simulink model "Glidescope_Flare_Simulink"  (R2024b)
settings: Solver=VariableStepAuto  StartTime=0.0  StopTime=250  RelTol=1e-3
values from neighbouring files (symbols this model uses):
  A_ac_p8 = A_long_p8(1:5,1:5)    [HA_ES_MainCode.m]    (also in PitchController.mat = [0 0 0.00013165266625 3.15369085605e-06 -4.69868043887e-21 2; glidescope.mat = [0 0 0.00013165266625 3.15369085605e-06 -4.69868043887e-21 2)
  B_ac_p8 = A_long_p8(1:5,6:7)    [HA_ES_MainCode.m]    (also in PitchController.mat = [0  0; 0  0; 0.00154396044469  -0.00453382205143; -9.4930881; glidescope.mat = [0  0; 0  0; 0.00154396044469  -0.00453382205143; -9.4930881)
  C_ac_p8 = C_long_p8(1:5,1:5)    [HA_ES_MainCode.m]    (also in PitchController.mat = [1 0 0 0 0 0 57.2957795131 0 0 0 0 0 ... (25 elements, 5x5)]; glidescope.mat = [1 0 0 0 0 0 57.2957795131 0 0 0 0 0 ... (25 elements, 5x5)])
  D_ac_p8 = C_long_p8(1:5,6:7)    [HA_ES_MainCode.m]    (also in PitchController.mat = [0  0; 0  0; 0  0; 0  0; 0  0]; glidescope.mat = [0  0; 0  0; 0  0; 0  0; 0  0])
  h0 = double(sol.h0)    [HA_ES_MainCode.m]    (also in PitchController.mat = 8.35170678627; glidescope.mat = 8.35170678627)
  hf = double(sol.hf)    [HA_ES_MainCode.m]    (also in PitchController.mat = 52.4513473104; glidescope.mat = 52.4513473104)
  Kv = 100    [HA_ES_MainCode.m]    (also in PitchController.mat; glidescope.mat)
  tau = double(sol.tau)    [HA_ES_MainCode.m]    (also in PitchController.mat = 0.497; glidescope.mat = 3.34068271451)
  xu_lo = [0 0 15000 0 0.0779375118365 0 500 0.0779375118365 0 0 0 0 ... (18 elements, 18x1)]    [PitchController.mat]    (also in glidescope.mat = [0 0 5000 0 0.182405640343 0 300 0.182405640343 0 0 0 0 ... )
libraries: slpidlib x1
settings Model: Creator=henryadam  LastModifiedBy=henryadam

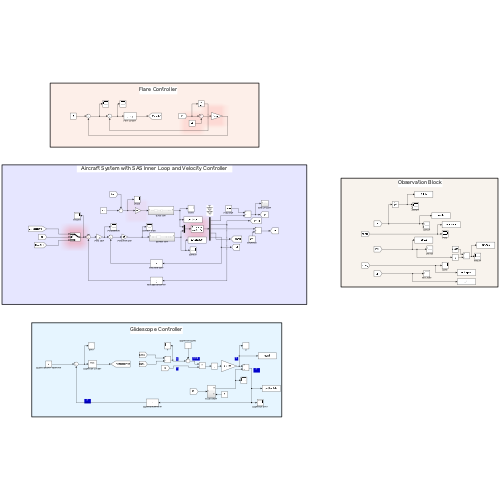
[thumbnail: Simulink's stored preview of the top-level diagram]
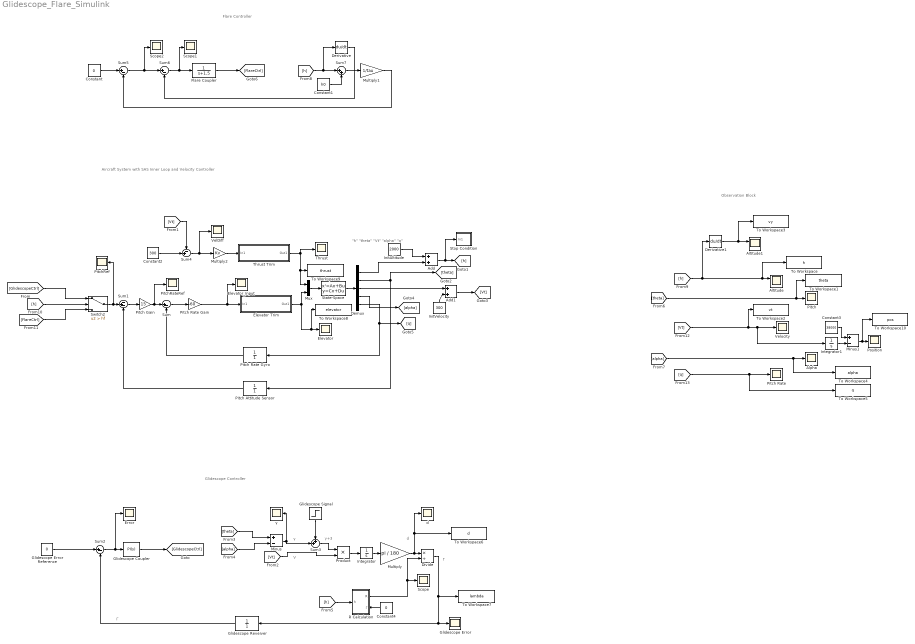
== system Glidescope_Flare_Simulink ==
  note: Aircraft System with SAS Inner Loop and Velocity Controller
  note: Glidescope Controller
  note: Flare Controller
  note: γ
  note: V
  note: Γ
  note: Γ
  note: "h"
      | "theta"
      | "Vt"
      | "alpha"
      | "q"
  note: γ+3
  note: d
  note: Observation Block
  Add : Sum
  Add1 : Sum
  Alpha : Scope
  Altitude : Scope  NumInputPorts=2
  Altitude1 : Scope  NumInputPorts=2
  Constant : Constant  Value=0
  Constant1 : Constant  Value=h0
  Constant2 : Constant  Value=300
  Constant3 : Constant  Value=38000
  Constant4 : Constant  Value=0
  Demux : Demux  Outputs=5
  Derivative : Derivative
  Derivative1 : Derivative
  Divide : Product  Inputs=*/
  Elevator : Scope
  Elevator Trim : Subsystem
  Elevator_Input : Scope
  Error : Scope
  Flare Coupler : TransferFcn  Denominator=[1 1.5]
  Glidescope Coupler : slpidlib/PID Controller  Controller=PI  Form=Parallel  TimeDomain=Continuous-time  UseExternalTs=off  SampleTime=-1  IntegratorMethod=Forward Euler  FilterMethod=Forward Euler  ControllerParametersSource=internal  P=17000  I=4000  UseKiTs=off  D=0  UseExternalDerivativeSource=off  N=100  UseFilter=on  TunerSelectOption=Transfer Function Based (PID Tuner App)  InitialConditionSource=internal  InitialConditionForIntegrator=0  InitialConditionForFilter=0  DifferentiatorICPrevScaledInput=0  ExternalReset=none  TrackingMode=off  Kt=1  LimitOutput=off  SatLimitsSource=internal  UpperSaturationLimit=inf  LowerSaturationLimit=-inf  LinearizeAsGain=on  AntiWindupMode=none  Kb=1  LimitIntegrator=off  UpperIntegratorSaturationLimit=inf  LowerIntegratorSaturationLimit=-inf  POutMin=[]  POutMax=[]  IOutMin=[]  IOutMax=[]  DOutMin=[]  DOutMax=[]  NOutMin=[]  NOutMax=[]  SumOutMin=[]  SumOutMax=[]  SaturationOutMin=[]  SaturationOutMax=[]  PParamMin=[]  PParamMax=[]  IParamMin=[]  IParamMax=[]  DParamMin=[]  DParamMax=[]  NParamMin=[]  NParamMax=[]  KbParamMin=[]  KbParamMax=[]  KtParamMin=[]  KtParamMax=[]  KbOutMin=[]  KbOutMax=[]  KtOutMin=[]  KtOutMax=[]  IntegratorOutMin=[]  IntegratorOutMax=[]  FilterOutMin=[]  FilterOutMax=[]  SumI1OutMin=[]  SumI1OutMax=[]  SumI2OutMin=[]  SumI2OutMax=[]  SumI3OutMin=[]  SumI3OutMax=[]  SumI4OutMin=[]  SumI4OutMax=[]  SumDOutMin=[]  SumDOutMax=[]  DifferentiatorOutMin=[]  DifferentiatorOutMax=[]  FilterDiffOutCoefMin=[]  FilterDiffOutCoefMax=[]  ReciprocalOutMin=[]  ReciprocalOutMax=[]  SumDenOutMin=[]  SumDenOutMax=[]  SumNumOutMin=[]  SumNumOutMax=[]  DivideOutMin=[]  DivideOutMax=[]  UdiffTsProdOutMin=[]  UdiffTsProdOutMax=[]  NTsProdOutMin=[]  NTsProdOutMax=[]  UintegralTsProdOutMin=[]  UintegralTsProdOutMax=[]  UngainTsProdOutMin=[]  UngainTsProdOutMax=[]  ClampingZeroOutDataTypeStr=Inherit: Inherit via back propagation  ClampingZeroOutMin=[]  ClampingZeroOutMax=[]  FilterDenConstantOutDataTypeStr=Inherit: Inherit via back propagation  FilterDenConstantOutMin=[]  FilterDenConstantOutMax=[]  PCopyOutDataTypeStr=Inherit: Inherit via back propagation  PCopyOutMin=[]  PCopyOutMax=[]  NCopyOutDataTypeStr=Inherit: Inherit via back propagation  NCopyOutMin=[]  NCopyOutMax=[]  IntegratorContinuousStateAttributes=''  IntegratorStateMustResolveToSignalObject=off  IntegratorRTWStateStorageClass=Auto  FilterContinuousStateAttributes=''  FilterStateMustResolveToSignalObject=off  FilterRTWStateStorageClass=Auto  ParallelPVariant=InternalParameters  IdealPVariant=Disabled  IVariant=InternalParameters  DVariant=Disabled  IntegratorVariant=Continuous  SatVariant=Disabled  AWVariant=Passthrough  PCopyVariant=Disabled  TRVariant=Disabled  FdbkBlocksVariant=Forward  IdealPFdbkVariant=Disabled  SatFdbkVariant=Disabled  DerivativeFilterVariant=Disabled  NVariant=Disabled  NCopyVariant=Disabled_SignalSpec  FilterICVariant=Disabled  IntegratorICVariant=InternalICs  ExternalResetVariant=Disabled  TRSumVariant=Passthrough  SumFdbkVariant=Disabled  SumVariant=Sum_PI  TsampFilterVariant=InternalTs  TsampNgainVariant=Passthrough  TsampIntegralVariant=Disabled_SignalSpec  ExternalSaturationOutDataTypeStr=Inherit: Same as second input  DerivativeSourceVariant=Disabled  PreIntVariant=InternalPreInt
  Glidescope Error : Scope
  Glidescope Error Reference : Constant  Value=0
  Glidescope Reveiver : TransferFcn  Denominator=[1]
  Glidescope Signal : Step  Time=10  After=3  SampleTime=0
  InitAltitude : Constant  Value=2000
  InitVelocity : Constant  Value=300
  Integrator : Integrator
  Integrator1 : Integrator
  Minus : Sum  Inputs=+-
  Minus1 : Sum  Inputs=+-
  Multiply : Gain  Gain=pi / 180
  Multiply1 : Gain  Gain=1/tau
  Multiply2 : Gain  Gain=Kv
  Mux : Mux  Inputs=2
  Pitch : Scope
  Pitch Attitude Sensor : TransferFcn  Denominator=[1]
  Pitch Gain : Gain  Gain=15
  Pitch Rate : Scope
  Pitch Rate Gain : Gain  Gain=-60
  Pitch Rate Gyro : TransferFcn  Denominator=[1]
  PitchRateRef : Scope
  PitchRef : Scope
  Position : Scope
  Product : Product
  R Calculation : Subsystem
      settings: PortSchema="{\"entries\":[{\"content\":{\"sides\":[{\"content\":{\"connectorIds\":[\"In1\"]},\"type\":\"ConnectorPlacement.EquallySpacedRectSide\",\"uuid\":\"a58ea4d3-e7df-4749-b01a-fc0a42cf2060\"},{\"content\":{\"connectorIds\":[\"Out1\",\"In2\"],\"side\":\"RIGHT\"},\"type\":\"ConnectorPlacement.EquallySpacedRectSide\",\"uuid\":\"27d5ff2b-4e59-4ac1-b665-58941cf67848\"},{\"content\":{\"side\":\"TOP\"},\"type\":\"ConnectorPlacement.EquallySpacedRectSide\",\"uuid\":\"e99417a1-aceb-4143-96dd-16120f62f201\"}]},\"type\":\"ConnectorPlacement.EquallySpacedConnector\",\"uuid\":\"f753324d-1728-43c1-b72b-a766f20cfffb\"}],\"packageUris\":[\"http://schema.mathworks.com/mf0/Connector/R2020b\"],\"version\":\"1.0\"}"
  Scope : Scope
  Scope1 : Scope
  Scope2 : Scope
  State-Space : StateSpace  A=A_ac_p8  B=B_ac_p8  C=C_ac_p8  D=D_ac_p8  InitialCondition=0
  Stop Condition : Subsystem
  Sum{,2,5..6} (4 alike) : Sum  Inputs=|+-
  Sum1 : Sum  Inputs=-+-
  Sum3 : Sum  Inputs=++|
  Sum4 : Sum  Inputs=-+|
  Sum7 : Sum  Inputs=|++
  Switch2 : Switch  Criteria=u2 > Threshold  Threshold=hf  SaturateOnIntegerOverflow=off  InputSameDT=off
  Thrust : Scope
  "Thrust Trim " : Subsystem
  To Workspace : ToWorkspace  VariableName=h  SaveFormat=Timeseries  SampleTime=-1
  To Workspace1 : ToWorkspace  VariableName=theta  SaveFormat=Timeseries  SampleTime=-1
  To Workspace10 : ToWorkspace  VariableName=pos  SaveFormat=Timeseries  SampleTime=-1
  To Workspace2 : ToWorkspace  VariableName=vt  SaveFormat=Timeseries  SampleTime=-1
  To Workspace3 : ToWorkspace  VariableName=vy  SaveFormat=Timeseries  SampleTime=-1
  To Workspace4 : ToWorkspace  VariableName=alpha  SaveFormat=Timeseries  SampleTime=-1
  To Workspace5 : ToWorkspace  VariableName=q  SaveFormat=Timeseries  SampleTime=-1
  To Workspace6 : ToWorkspace  VariableName=d  SaveFormat=Timeseries  SampleTime=-1
  To Workspace7 : ToWorkspace  VariableName=lambda  SaveFormat=Timeseries  SampleTime=-1
  To Workspace8 : ToWorkspace  VariableName=elevator  SaveFormat=Timeseries  SampleTime=-1
  To Workspace9 : ToWorkspace  VariableName=thrust  SaveFormat=Timeseries  SampleTime=-1
  VelDiff : Scope
  "Velocity " : Scope
  d : Scope
  γ : Scope
  wires:
  Sum/1 -> Pitch Rate Gain/1
  Pitch Rate Gyro/1 -> Sum/2
  Pitch Gain/1 -> PitchRateRef/1, Sum/1
  Sum1/1 -> Pitch Gain/1
  Pitch Attitude Sensor/1 -> Sum1/3
  Multiply/1 -> To Workspace6/1, d/1, Divide/1
  Divide/1 -> To Workspace7/1, Glidescope Error/1, Glidescope Reveiver/1
  Sum2/1 -> Error/1, Glidescope Coupler/1
  Pitch Rate Gain/1 -> Elevator Trim/1(In1), Elevator_Input/1
  Elevator Trim/1(Out1) -> Mux/2, To Workspace8/1, Elevator/1
  "Thrust Trim "/1(Out1) -> To Workspace9/1, Mux/1, Thrust/1
  Mux/1 -> State-Space/1
  State-Space/1 -> Demux/1
  Glidescope Error Reference/1 -> Sum2/1
  Minus/1 -> Sum3/2, γ/1
  Glidescope Signal/1 -> Sum3/1
  Sum3/1 -> Product/1
  Sum6/1 -> Scope1/1, Flare Coupler/1
  [h] -> Sum7/1, Derivative/1
  Derivative/1 -> Sum6/2
  Multiply1/1 -> Sum5/2
  Sum4/1 -> VelDiff/1, Multiply2/1
  Constant2/1 -> Sum4/2
  Sum7/1 -> Multiply1/1
  Constant1/1 -> Sum7/2
  [h] -> Derivative1/1, To Workspace/1, Altitude/1
  [theta] -> To Workspace1/1, Pitch/1
  [q] -> To Workspace5/1, Pitch Rate/1
  [Vt] -> To Workspace2/1, Integrator1/1, "Velocity "/1
  [alpha] -> To Workspace4/1, Alpha/1
  Multiply2/1 -> "Thrust Trim "/1(In1)
  Integrator/1 -> Multiply/1
  Product/1 -> Integrator/1
  Constant4/1 -> R Calculation/2(Γ)
  Switch2/1 -> PitchRef/1, Sum1/2
  Glidescope Reveiver/1 -> Sum2/2
  R Calculation/1(R) -> Divide/2, Scope/1
  [Vt] -> Sum4/1
  [Vt] -> Product/2
  [theta] -> Minus/1
  [alpha] -> Minus/2
  [h] -> R Calculation/1(h)
  Demux/2 -> [theta], Pitch Attitude Sensor/1
  Demux/5 -> [q], Pitch Rate Gyro/1
  Demux/4 -> [alpha]
  Glidescope Coupler/1 -> [GlidescopeCtrl]
  [GlidescopeCtrl] -> Switch2/1
  [h] -> Switch2/2
  [FlareCtrl] -> Switch2/3
  Flare Coupler/1 -> [FlareCtrl]
  Add/1 -> Stop Condition/1(In1), [h]
  Demux/1 -> Add/2
  InitAltitude/1 -> Add/1
  Add1/1 -> [Vt]
  Demux/3 -> Add1/1
  InitVelocity/1 -> Add1/2
  Constant/1 -> Sum5/1
  Sum5/1 -> Scope2/1, Sum6/1
  Derivative1/1 -> To Workspace3/1, Altitude1/1
  Integrator1/1 -> Minus1/2
  Constant3/1 -> Minus1/1
  Minus1/1 -> To Workspace10/1, Position/1

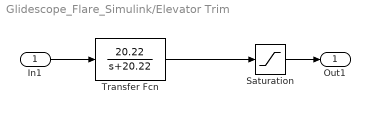
== system Glidescope_Flare_Simulink/Elevator Trim ==
  In1 : Inport
  Saturation : Saturate  UpperLimit=25 - xu_lo(14)  LowerLimit=-25 - xu_lo(14)
  Transfer Fcn : TransferFcn  Numerator=[0, 20.22]  Denominator=[1 20.22]
  Out1 : Outport
  wires:
  In1/1 -> Transfer Fcn/1
  Transfer Fcn/1 -> Saturation/1
  Saturation/1 -> Out1/1

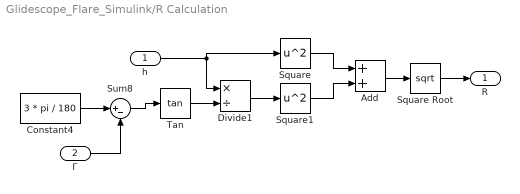
== system Glidescope_Flare_Simulink/R Calculation ==
  h : Inport
  Γ : Inport  Port=2
  Add : Sum
  Constant4 : Constant  Value=3 * pi / 180
  Divide1 : Product  Inputs=*/
  Square : Math  Operator=square
  Square Root : Sqrt
  Square1 : Math  Operator=square
  Sum8 : Sum  Inputs=|+-
  Tan : Trigonometry  Operator=tan
  R : Outport
  wires:
  Sum8/1 -> Tan/1
  Divide1/1 -> Square1/1
  Add/1 -> Square Root/1
  Constant4/1 -> Sum8/1
  Γ/1 -> Sum8/2
  Square/1 -> Add/1
  h/1 -> Square/1, Divide1/1
  Square Root/1 -> R/1
  Square1/1 -> Add/2
  Tan/1 -> Divide1/2

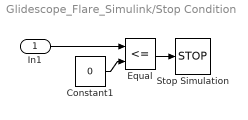
== system Glidescope_Flare_Simulink/Stop Condition ==
  In1 : Inport
  Constant1 : Constant  Value=0
  Equal : RelationalOperator  Operator=<=  OutDataTypeStr=boolean  RndMeth=Simplest  InputSameDT=off
  Stop Simulation : Stop
  wires:
  In1/1 -> Equal/1
  Constant1/1 -> Equal/2
  Equal/1 -> Stop Simulation/1

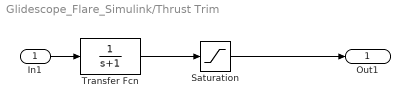
== system Glidescope_Flare_Simulink/Thrust Trim  ==
  In1 : Inport
  Saturation : Saturate  UpperLimit=19000 - xu_lo(13)  LowerLimit=1000 - xu_lo(13)
  Transfer Fcn : TransferFcn  Denominator=[1 1]
  Out1 : Outport
  wires:
  In1/1 -> Transfer Fcn/1
  Transfer Fcn/1 -> Saturation/1
  Saturation/1 -> Out1/1
